simulink model "Model_TranslationEngine64"  (R2022b)
settings: Solver=FixedStepDiscrete  StartTime=0.0  StopTime=5  RelTol=1e-3  EnableMultiTasking=on
InitFcn:
  | % Initialize model
  | ModelSettings=BTConfig.GetModelSettings();
  | 
  | ModelSettings.Validate();
  | 
  | ModelInit;
  | 
  | 
  | % load library data
  | GainLibrary_data;
  | % Load saved values from partition process
  | CapturedConstMask.LoadMapFromFile(bdroot)
StartFcn:
  | % make sure all the simulated RTC requests are found
  | %RTC_SIM_OBJ.ValidateREQs();
undefined symbols (not defined in the file or in its folder): AA, BPLP, Column, NumHFRefBPF, NumHFRefLPF, NumMusicChannels, Row, VolumeMuteConfig
libraries: TuneVar x925, TOP x490, FeaturePath x111, CapturedConstLib x52
(part 16 of 34)

== system Model_TranslationEngine64/NEAR/Near1p1/VolumeMute/VolMuteCh2/Mute/MuteControl ==
  FeaturePath : FeaturePath/FeaturePath  FeatureName=Ann2Mute  IsGroup=off  GroupNumber=-1  IsModule=off  TriggerInit=[180 39 295 146]
      settings: SourceProductName=Bose Talaria
  TuneVarRampTime : Subsystem  Description=|  mask(Talaria Trivial Tune TOP){TriggerInit=[295 232 465 288], TopName=RampTime, TuneName=RampTime, DataTypeOut=single, MaskValue=Config.DefaultRampTimeMsec, TunabilityNumber=1, MinValue=1, MaxValue=100000, BankNumber=0, PreOverlay=false, PostOverlay=false, UseSameName=on}
      | Specifies the default value of ramp time for the Mute or Unmute operation.
      | Used only when the RTC message does not contain either ramp rate or ramp time.
      mask prompts: TriggerInit "Hidden: MoveFcn redraw"; TopName "Name:"; TuneName "Name of TuneVar:"; DataTypeOut "Data type:"; MaskValue "Default Value:"; TunabilityNumber "Tunability:"; MinValue "Min Value:"; MaxValue "Max Value:"; BankNumber "Target memory bank number:"; PreOverlay "Requires pre-overlay action:"; PostOverlay "Requires post-overlay action:"; UseSameName "Use same name for tune variable and TOP"
      mask help: The TuneTOP block encapsultes a Target Overlay Parameter, a Tune Variable, and a Trivial Translation between them.
      mask init:
      | [ok,activeTopPath,activeTunePath] = TuneTOP_Mask.Init(gcbh);
      settings: MoveFcn=TuneTOP_Mask.CB_TriggerInit(gcbh);
      mask Callback TriggerInit: TuneTOP_Mask.CB_TriggerInit(gcbh);
      mask TypeOptions TopName: TOP/TopName
      mask TypeOptions TuneName: Tune Variable/TuneName
      mask TypeOptions DataTypeOut: TOP/DataTypeOut
      mask TypeOptions MaskValue: Tune Variable/MaskValue
      mask TypeOptions TunabilityNumber: Tune Variable/TunabilityNumber
      mask Callback TunabilityNumber: TuneVarMask.CB_TunabilityNumber(gcbh);
      mask TypeOptions MinValue: Tune Variable/MinValue
      mask TypeOptions MaxValue: Tune Variable/MaxValue
      mask TypeOptions BankNumber: TOP/BankNumber
      mask TypeOptions PreOverlay: TOP/PreOverlay
      mask TypeOptions PostOverlay: TOP/PostOverlay
      mask Callback UseSameName: TuneTOP_Mask.CB_UseSameName(gcbh);
      mask DialogControl toolPanel Prompt: Tuning Tool Hints
      mask DialogControl DescriptionGroup Prompt: Description
      mask DialogControl EditDescription Prompt: Edit Description
      mask DialogControl EditDescription Callback: TuneTOP_Mask.CB_EditDescription(gcbh);
      mask DialogControl TunabilityText Prompt: Easy: Changes nearly every tuning.
      mask DialogControl AdvancedPanel Prompt: Advanced
      mask DialogControl ConvertToFullTranslation Prompt: Irreversible conversion to full translation
      mask DialogControl ConvertToFullTranslation Callback: TuneTOP_Mask.CB_ConvertToFullTranslation(gcbh);
      mask DialogControl ErrorContainer Prompt: Error Messages
      mask Display:
      | % retrieve icon definition
      | [path,w,h] = TuneTOP_Mask.Icon();
      | 
      | % retrieve the block's pixel size
      | pos = get(gcbh,'position');
      | bw = pos(3) - pos(1);
      | bh = pos(4) - pos(2);
      | 
      | % draw centered icon
      | xAdj = bw/2 - w/2 + 5;
      | yAdj = bh/2 - h/2 + 4;
      | for i=1:length(path)
      | 	patch(path(i).x+xAdj, path(i).y+yAdj, path(i).rgb);
      | end
      | 
      | % show the top name or an X
      | if (exist('ok','var') && ok)
      | 	text(bw*0.5, bh*0.2, activeTopPath, 'horizontalAlignment', 'center');
      | 	patch(0,0,[1 1 1]);
      | 	patch(bw,bh,[1 1 1]);
      | else
      | 	tx=bw*0.03;
      | 	ty=bh*0.03;
      | 	patch([0 tx bw bw-tx], [ty 0 bh-ty bh], [1 0 0]);
      | 	patch([0 bw-tx bw tx], [bh-ty 0 ty bh], [1 0 0]);
      | end

== system Model_TranslationEngine64/NEAR/Near1p1/VolumeMute/VolMuteCh2/Volume/TuneVarRampRate ==
  TOP : TOP/TOP  TriggerInit=[440 20 585 80]  TopName=RampRate  DataTypeOut=single  BankNumber=BankNumber  PreOverlay=PreOverlay  PostOverlay=PostOverlay  Role=Automatic
      settings: SourceProductName=Bose Talaria
  TrivialTranslation : TuneVar/TrivialTranslation  TriggerInit=[300 28 350 72]
      settings: SourceProductName=Bose Talaria
  Tune Variable : TuneVar/TuneVar  TuneName=RampRate  SpecifyMaxSize=off  VariableDim=1 (Row)  MaxSize=[1 1]  TunabilityNumber=2  MinValue=MinValue  MaxValue=MaxValue  TriggerInit=[20 25 190 75]  MaskValue=MaskValue
      settings: SourceProductName=Bose Talaria
  wires:
  Tune Variable/1 -> TrivialTranslation/1  "RampRate"
  TrivialTranslation/1 -> TOP/1

== system Model_TranslationEngine64/NEAR/Near1p1/VolumeMute/VolMuteCh2/Volume/TuneVarRampTime ==
  TOP : TOP/TOP  TriggerInit=[440 20 585 80]  TopName=RampTime  DataTypeOut=single  BankNumber=BankNumber  PreOverlay=PreOverlay  PostOverlay=PostOverlay  Role=Automatic
      settings: SourceProductName=Bose Talaria
  TrivialTranslation : TuneVar/TrivialTranslation  TriggerInit=[300 28 350 72]
      settings: SourceProductName=Bose Talaria
  Tune Variable : TuneVar/TuneVar  TuneName=RampTime  SpecifyMaxSize=off  VariableDim=1 (Row)  MaxSize=[1 1]  TunabilityNumber=1  MinValue=MinValue  MaxValue=MaxValue  TriggerInit=[20 25 190 75]  MaskValue=MaskValue
      settings: SourceProductName=Bose Talaria
  wires:
  Tune Variable/1 -> TrivialTranslation/1  "RampTime"
  TrivialTranslation/1 -> TOP/1

== system Model_TranslationEngine64/NEAR/Near1p1/VolumeMute/VolMuteCh3/Ann3NonEntGainCalc/TuneTOP ==
  TOP : TOP/TOP  TriggerInit=[440 20 585 80]  TopName=VncThresh  DataTypeOut=single  BankNumber=BankNumber  PreOverlay=PreOverlay  PostOverlay=PostOverlay  Role=Automatic
      settings: SourceProductName=Bose Talaria
  TrivialTranslation : TuneVar/TrivialTranslation  TriggerInit=[300 28 350 72]
      settings: SourceProductName=Bose Talaria
  Tune Variable : TuneVar/TuneVar  TuneName=VncThresh  SpecifyMaxSize=off  VariableDim=1 (Row)  MaxSize=[1 1]  TunabilityNumber=1  MinValue=MinValue  MaxValue=MaxValue  TriggerInit=[20 25 190 75]  MaskValue=MaskValue
      settings: SourceProductName=Bose Talaria
  wires:
  Tune Variable/1 -> TrivialTranslation/1  "VncThresh"
  TrivialTranslation/1 -> TOP/1

== system Model_TranslationEngine64/NEAR/Near1p1/VolumeMute/VolMuteCh3/Ann3NonEntGainCalc/TuneTOP1 ==
  TOP : TOP/TOP  TriggerInit=[440 20 585 80]  TopName=VncSlope  DataTypeOut=single  BankNumber=BankNumber  PreOverlay=PreOverlay  PostOverlay=PostOverlay  Role=Automatic
      settings: SourceProductName=Bose Talaria
  TrivialTranslation : TuneVar/TrivialTranslation  TriggerInit=[300 28 350 72]
      settings: SourceProductName=Bose Talaria
  Tune Variable : TuneVar/TuneVar  TuneName=VncSlope  SpecifyMaxSize=off  VariableDim=1 (Row)  MaxSize=[1 1]  TunabilityNumber=1  MinValue=MinValue  MaxValue=MaxValue  TriggerInit=[20 25 190 75]  MaskValue=MaskValue
      settings: SourceProductName=Bose Talaria
  wires:
  Tune Variable/1 -> TrivialTranslation/1  "VncSlope"
  TrivialTranslation/1 -> TOP/1

== system Model_TranslationEngine64/NEAR/Near1p1/VolumeMute/VolMuteCh3/Ann3NonEntGainCalc/TuneTOP2 ==
  TOP : TOP/TOP  TriggerInit=[440 20 585 80]  TopName=MaxBoost  DataTypeOut=single  BankNumber=BankNumber  PreOverlay=PreOverlay  PostOverlay=PostOverlay  Role=Automatic
      settings: SourceProductName=Bose Talaria
  TrivialTranslation : TuneVar/TrivialTranslation  TriggerInit=[300 28 350 72]
      settings: SourceProductName=Bose Talaria
  Tune Variable : TuneVar/TuneVar  TuneName=MaxBoost  SpecifyMaxSize=off  VariableDim=1 (Row)  MaxSize=[1 1]  TunabilityNumber=1  MinValue=MinValue  MaxValue=MaxValue  TriggerInit=[20 25 190 75]  MaskValue=MaskValue
      settings: SourceProductName=Bose Talaria
  wires:
  Tune Variable/1 -> TrivialTranslation/1  "MaxBoost"
  TrivialTranslation/1 -> TOP/1

== system Model_TranslationEngine64/NEAR/Near1p1/VolumeMute/VolMuteCh3/Ann3NonEntGainCalc/TuneTOP3 ==
  TOP : TOP/TOP  TriggerInit=[440 20 585 80]  TopName=NoiseOverRide  DataTypeOut=single  BankNumber=BankNumber  PreOverlay=PreOverlay  PostOverlay=PostOverlay  Role=Automatic
      settings: SourceProductName=Bose Talaria
  TrivialTranslation : TuneVar/TrivialTranslation  TriggerInit=[300 28 350 72]
      settings: SourceProductName=Bose Talaria
  Tune Variable : TuneVar/TuneVar  TuneName=NoiseOverRide  SpecifyMaxSize=off  VariableDim=1 (Row)  MaxSize=[1 1]  TunabilityNumber=1  MinValue=MinValue  MaxValue=MaxValue  TriggerInit=[20 25 190 75]  MaskValue=MaskValue
      settings: SourceProductName=Bose Talaria
  wires:
  Tune Variable/1 -> TrivialTranslation/1  "NoiseOverRide"
  TrivialTranslation/1 -> TOP/1

== system Model_TranslationEngine64/NEAR/Near1p1/VolumeMute/VolMuteCh3/Ann3NonEntGainCalc/TuneTOP4 ==
  TOP : TOP/TOP  TriggerInit=[440 20 585 80]  TopName=NoiseOverRideFlag  DataTypeOut=single  BankNumber=BankNumber  PreOverlay=PreOverlay  PostOverlay=PostOverlay  Role=Automatic
      settings: SourceProductName=Bose Talaria
  TrivialTranslation : TuneVar/TrivialTranslation  TriggerInit=[300 28 350 72]
      settings: SourceProductName=Bose Talaria
  Tune Variable : TuneVar/TuneVar  TuneName=NoiseOverRideFlag  SpecifyMaxSize=off  VariableDim=1 (Row)  MaxSize=[1 1]  TunabilityNumber=1  MinValue=MinValue  MaxValue=MaxValue  TriggerInit=[20 25 190 75]  MaskValue=MaskValue
      settings: SourceProductName=Bose Talaria
  wires:
  Tune Variable/1 -> TrivialTranslation/1  "NoiseOverRideFlag"
  TrivialTranslation/1 -> TOP/1

== system Model_TranslationEngine64/NEAR/Near1p1/VolumeMute/VolMuteCh3/Ann3NonEntGainCalc/TuneTOP5 ==
  TOP : TOP/TOP  TriggerInit=[440 20 585 80]  TopName=BoostOverRide  DataTypeOut=single  BankNumber=BankNumber  PreOverlay=PreOverlay  PostOverlay=PostOverlay  Role=Automatic
      settings: SourceProductName=Bose Talaria
  TrivialTranslation : TuneVar/TrivialTranslation  TriggerInit=[300 28 350 72]
      settings: SourceProductName=Bose Talaria
  Tune Variable : TuneVar/TuneVar  TuneName=BoostOverRide  SpecifyMaxSize=off  VariableDim=1 (Row)  MaxSize=[1 1]  TunabilityNumber=1  MinValue=MinValue  MaxValue=MaxValue  TriggerInit=[20 25 190 75]  MaskValue=MaskValue
      settings: SourceProductName=Bose Talaria
  wires:
  Tune Variable/1 -> TrivialTranslation/1  "BoostOverRide"
  TrivialTranslation/1 -> TOP/1

== system Model_TranslationEngine64/NEAR/Near1p1/VolumeMute/VolMuteCh3/Ann3NonEntGainCalc/TuneTOP6 ==
  TOP : TOP/TOP  TriggerInit=[440 20 585 80]  TopName=BoostOverRideFlag  DataTypeOut=single  BankNumber=BankNumber  PreOverlay=PreOverlay  PostOverlay=PostOverlay  Role=Automatic
      settings: SourceProductName=Bose Talaria
  TrivialTranslation : TuneVar/TrivialTranslation  TriggerInit=[300 28 350 72]
      settings: SourceProductName=Bose Talaria
  Tune Variable : TuneVar/TuneVar  TuneName=BoostOverRideFlag  SpecifyMaxSize=off  VariableDim=1 (Row)  MaxSize=[1 1]  TunabilityNumber=1  MinValue=MinValue  MaxValue=MaxValue  TriggerInit=[20 25 190 75]  MaskValue=MaskValue
      settings: SourceProductName=Bose Talaria
  wires:
  Tune Variable/1 -> TrivialTranslation/1  "BoostOverRideFlag"
  TrivialTranslation/1 -> TOP/1

== system Model_TranslationEngine64/NEAR/Near1p1/VolumeMute/VolMuteCh3/Ann3NonEntGainCalc/TuneTOP7 ==
  TOP : TOP/TOP  TriggerInit=[440 20 585 80]  TopName=VncEnableTuneVar  DataTypeOut=single  BankNumber=BankNumber  PreOverlay=PreOverlay  PostOverlay=PostOverlay  Role=Automatic
      settings: SourceProductName=Bose Talaria
  TrivialTranslation : TuneVar/TrivialTranslation  TriggerInit=[300 28 350 72]
      settings: SourceProductName=Bose Talaria
  Tune Variable : TuneVar/TuneVar  TuneName=VncEnableTuneVar  SpecifyMaxSize=off  VariableDim=1 (Row)  MaxSize=[1 1]  TunabilityNumber=1  MinValue=MinValue  MaxValue=MaxValue  TriggerInit=[20 25 190 75]  MaskValue=MaskValue
      settings: SourceProductName=Bose Talaria
  wires:
  Tune Variable/1 -> TrivialTranslation/1  "VncEnableTuneVar"
  TrivialTranslation/1 -> TOP/1

== system Model_TranslationEngine64/NEAR/Near1p1/VolumeMute/VolMuteCh3/Ann3NonEntGainCalc/TuneTOP8 ==
  TranslateTrigger : TuneVar/TranslateTrigger  TriggerInit=[306 -100 344 -45]
      settings: SourceProductName=Bose Talaria
  den : TOP/TOP  TriggerInit=[450 90 595 150]  TopName=Den  DataTypeOut=single  BankNumber=0  PreOverlay=false  PostOverlay=false  Role=Automatic
      settings: SourceProductName=Bose Talaria
  num : TOP/TOP  TriggerInit=[450 -45 595 15]  TopName=Num  DataTypeOut=single  BankNumber=0  PreOverlay=false  PostOverlay=false  Role=Automatic
      settings: SourceProductName=Bose Talaria
  translation : MATLAB Function  TreatAsAtomicUnit=on  mask{L=Config.FrameSize, Fd=Config.Fd}
  tuneVARTau : TuneVar/TuneVar  TuneName=Tau  SpecifyMaxSize=off  VariableDim=1 (Row)  MaxSize=[1 1]  TunabilityNumber=1  MinValue=[]  MaxValue=[]  TriggerInit=[-70 25 100 75]  MaskValue=Config.DefaultTau
      settings: SourceProductName=Bose Talaria
  wires:
  tuneVARTau/1 -> translation/1(tau)  "Tau"
  TranslateTrigger/1 -> translation/Trigger
  translation/2(Den) -> den/1
  translation/1(Num) -> num/1

== system Model_TranslationEngine64/NEAR/Near1p1/VolumeMute/VolMuteCh3/Ann3NonEntGainCalc/vncSignal ==
  TuneTOP : Subsystem  mask(Talaria Trivial Tune TOP){TriggerInit=[50 -8 220 48], TopName=MinVncSignal, TuneName=MinVncSignal, DataTypeOut=single, MaskValue=Config.DefaultMinVncSignal, TunabilityNumber=1, MinValue=[], MaxValue=[], BankNumber=0, PreOverlay=false, PostOverlay=false, UseSameName=on}
      mask prompts: TriggerInit "Hidden: MoveFcn redraw"; TopName "Name:"; TuneName "Name of TuneVar:"; DataTypeOut "Data type:"; MaskValue "Default Value:"; TunabilityNumber "Tunability:"; MinValue "Min Value:"; MaxValue "Max Value:"; BankNumber "Target memory bank number:"; PreOverlay "Requires pre-overlay action:"; PostOverlay "Requires post-overlay action:"; UseSameName "Use same name for tune variable and TOP"
      mask help: The TuneTOP block encapsultes a Target Overlay Parameter, a Tune Variable, and a Trivial Translation between them.
      mask init:
      | [ok,activeTopPath,activeTunePath] = TuneTOP_Mask.Init(gcbh);
      settings: MoveFcn=TuneTOP_Mask.CB_TriggerInit(gcbh);
      mask Callback TriggerInit: TuneTOP_Mask.CB_TriggerInit(gcbh);
      mask TypeOptions TopName: TOP/TopName
      mask TypeOptions TuneName: Tune Variable/TuneName
      mask TypeOptions DataTypeOut: TOP/DataTypeOut
      mask TypeOptions MaskValue: Tune Variable/MaskValue
      mask TypeOptions TunabilityNumber: Tune Variable/TunabilityNumber
      mask Callback TunabilityNumber: TuneVarMask.CB_TunabilityNumber(gcbh);
      mask TypeOptions MinValue: Tune Variable/MinValue
      mask TypeOptions MaxValue: Tune Variable/MaxValue
      mask TypeOptions BankNumber: TOP/BankNumber
      mask TypeOptions PreOverlay: TOP/PreOverlay
      mask TypeOptions PostOverlay: TOP/PostOverlay
      mask Callback UseSameName: TuneTOP_Mask.CB_UseSameName(gcbh);
      mask DialogControl toolPanel Prompt: Tuning Tool Hints
      mask DialogControl DescriptionGroup Prompt: Description
      mask DialogControl EditDescription Prompt: Edit Description
      mask DialogControl EditDescription Callback: TuneTOP_Mask.CB_EditDescription(gcbh);
      mask DialogControl TunabilityText Prompt: Easy: Changes nearly every tuning.
      mask DialogControl AdvancedPanel Prompt: Advanced
      mask DialogControl ConvertToFullTranslation Prompt: Irreversible conversion to full translation
      mask DialogControl ConvertToFullTranslation Callback: TuneTOP_Mask.CB_ConvertToFullTranslation(gcbh);
      mask DialogControl ErrorContainer Prompt: Error Messages
      mask Display:
      | % retrieve icon definition
      | [path,w,h] = TuneTOP_Mask.Icon();
      | 
      | % retrieve the block's pixel size
      | pos = get(gcbh,'position');
      | bw = pos(3) - pos(1);
      | bh = pos(4) - pos(2);
      | 
      | % draw centered icon
      | xAdj = bw/2 - w/2 + 5;
      | yAdj = bh/2 - h/2 + 4;
      | for i=1:length(path)
      | 	patch(path(i).x+xAdj, path(i).y+yAdj, path(i).rgb);
      | end
      | 
      | % show the top name or an X
      | if (exist('ok','var') && ok)
      | 	text(bw*0.5, bh*0.2, activeTopPath, 'horizontalAlignment', 'center');
      | 	patch(0,0,[1 1 1]);
      | 	patch(bw,bh,[1 1 1]);
      | else
      | 	tx=bw*0.03;
      | 	ty=bh*0.03;
      | 	patch([0 tx bw bw-tx], [ty 0 bh-ty bh], [1 0 0]);
      | 	patch([0 bw-tx bw tx], [bh-ty 0 ty bh], [1 0 0]);
      | end
  TuneTOP1 : Subsystem  mask(Talaria Trivial Tune TOP){TriggerInit=[40 142 210 198], TopName=MaxSpl, TuneName=MaxSpl, DataTypeOut=single, MaskValue=Config.DefaultMaxSpl, TunabilityNumber=1, MinValue=[], MaxValue=[], BankNumber=0, PreOverlay=false, PostOverlay=false, UseSameName=on}
      mask prompts: TriggerInit "Hidden: MoveFcn redraw"; TopName "Name:"; TuneName "Name of TuneVar:"; DataTypeOut "Data type:"; MaskValue "Default Value:"; TunabilityNumber "Tunability:"; MinValue "Min Value:"; MaxValue "Max Value:"; BankNumber "Target memory bank number:"; PreOverlay "Requires pre-overlay action:"; PostOverlay "Requires post-overlay action:"; UseSameName "Use same name for tune variable and TOP"
      mask help: The TuneTOP block encapsultes a Target Overlay Parameter, a Tune Variable, and a Trivial Translation between them.
      mask init:
      | [ok,activeTopPath,activeTunePath] = TuneTOP_Mask.Init(gcbh);
      settings: MoveFcn=TuneTOP_Mask.CB_TriggerInit(gcbh);
      mask Callback TriggerInit: TuneTOP_Mask.CB_TriggerInit(gcbh);
      mask TypeOptions TopName: TOP/TopName
      mask TypeOptions TuneName: Tune Variable/TuneName
      mask TypeOptions DataTypeOut: TOP/DataTypeOut
      mask TypeOptions MaskValue: Tune Variable/MaskValue
      mask TypeOptions TunabilityNumber: Tune Variable/TunabilityNumber
      mask Callback TunabilityNumber: TuneVarMask.CB_TunabilityNumber(gcbh);
      mask TypeOptions MinValue: Tune Variable/MinValue
      mask TypeOptions MaxValue: Tune Variable/MaxValue
      mask TypeOptions BankNumber: TOP/BankNumber
      mask TypeOptions PreOverlay: TOP/PreOverlay
      mask TypeOptions PostOverlay: TOP/PostOverlay
      mask Callback UseSameName: TuneTOP_Mask.CB_UseSameName(gcbh);
      mask DialogControl toolPanel Prompt: Tuning Tool Hints
      mask DialogControl DescriptionGroup Prompt: Description
      mask DialogControl EditDescription Prompt: Edit Description
      mask DialogControl EditDescription Callback: TuneTOP_Mask.CB_EditDescription(gcbh);
      mask DialogControl TunabilityText Prompt: Easy: Changes nearly every tuning.
      mask DialogControl AdvancedPanel Prompt: Advanced
      mask DialogControl ConvertToFullTranslation Prompt: Irreversible conversion to full translation
      mask DialogControl ConvertToFullTranslation Callback: TuneTOP_Mask.CB_ConvertToFullTranslation(gcbh);
      mask DialogControl ErrorContainer Prompt: Error Messages
      mask Display:
      | % retrieve icon definition
      | [path,w,h] = TuneTOP_Mask.Icon();
      | 
      | % retrieve the block's pixel size
      | pos = get(gcbh,'position');
      | bw = pos(3) - pos(1);
      | bh = pos(4) - pos(2);
      | 
      | % draw centered icon
      | xAdj = bw/2 - w/2 + 5;
      | yAdj = bh/2 - h/2 + 4;
      | for i=1:length(path)
      | 	patch(path(i).x+xAdj, path(i).y+yAdj, path(i).rgb);
      | end
      | 
      | % show the top name or an X
      | if (exist('ok','var') && ok)
      | 	text(bw*0.5, bh*0.2, activeTopPath, 'horizontalAlignment', 'center');
      | 	patch(0,0,[1 1 1]);
      | 	patch(bw,bh,[1 1 1]);
      | else
      | 	tx=bw*0.03;
      | 	ty=bh*0.03;
      | 	patch([0 tx bw bw-tx], [ty 0 bh-ty bh], [1 0 0]);
      | 	patch([0 bw-tx bw tx], [bh-ty 0 ty bh], [1 0 0]);
      | end

== system Model_TranslationEngine64/NEAR/Near1p1/VolumeMute/VolMuteCh3/Ann3NonEntVncApplied/nonentVNCApplied_subsystem ==
  TuneTOP : Subsystem

== system Model_TranslationEngine64/NEAR/Near1p1/VolumeMute/VolMuteCh3/Mute/MuteControl ==
  FeaturePath : FeaturePath/FeaturePath  FeatureName=Ann3Mute  IsGroup=off  GroupNumber=-1  IsModule=off  TriggerInit=[180 39 295 146]
      settings: SourceProductName=Bose Talaria
  TuneVarRampTime : Subsystem  Description=|  mask(Talaria Trivial Tune TOP){TriggerInit=[295 232 465 288], TopName=RampTime, TuneName=RampTime, DataTypeOut=single, MaskValue=Config.DefaultRampTimeMsec, TunabilityNumber=1, MinValue=1, MaxValue=100000, BankNumber=0, PreOverlay=false, PostOverlay=false, UseSameName=on}
      | Specifies the default value of ramp time for the Mute or Unmute operation.
      | Used only when the RTC message does not contain either ramp rate or ramp time.
      mask prompts: TriggerInit "Hidden: MoveFcn redraw"; TopName "Name:"; TuneName "Name of TuneVar:"; DataTypeOut "Data type:"; MaskValue "Default Value:"; TunabilityNumber "Tunability:"; MinValue "Min Value:"; MaxValue "Max Value:"; BankNumber "Target memory bank number:"; PreOverlay "Requires pre-overlay action:"; PostOverlay "Requires post-overlay action:"; UseSameName "Use same name for tune variable and TOP"
      mask help: The TuneTOP block encapsultes a Target Overlay Parameter, a Tune Variable, and a Trivial Translation between them.
      mask init:
      | [ok,activeTopPath,activeTunePath] = TuneTOP_Mask.Init(gcbh);
      settings: MoveFcn=TuneTOP_Mask.CB_TriggerInit(gcbh);
      mask Callback TriggerInit: TuneTOP_Mask.CB_TriggerInit(gcbh);
      mask TypeOptions TopName: TOP/TopName
      mask TypeOptions TuneName: Tune Variable/TuneName
      mask TypeOptions DataTypeOut: TOP/DataTypeOut
      mask TypeOptions MaskValue: Tune Variable/MaskValue
      mask TypeOptions TunabilityNumber: Tune Variable/TunabilityNumber
      mask Callback TunabilityNumber: TuneVarMask.CB_TunabilityNumber(gcbh);
      mask TypeOptions MinValue: Tune Variable/MinValue
      mask TypeOptions MaxValue: Tune Variable/MaxValue
      mask TypeOptions BankNumber: TOP/BankNumber
      mask TypeOptions PreOverlay: TOP/PreOverlay
      mask TypeOptions PostOverlay: TOP/PostOverlay
      mask Callback UseSameName: TuneTOP_Mask.CB_UseSameName(gcbh);
      mask DialogControl toolPanel Prompt: Tuning Tool Hints
      mask DialogControl DescriptionGroup Prompt: Description
      mask DialogControl EditDescription Prompt: Edit Description
      mask DialogControl EditDescription Callback: TuneTOP_Mask.CB_EditDescription(gcbh);
      mask DialogControl TunabilityText Prompt: Easy: Changes nearly every tuning.
      mask DialogControl AdvancedPanel Prompt: Advanced
      mask DialogControl ConvertToFullTranslation Prompt: Irreversible conversion to full translation
      mask DialogControl ConvertToFullTranslation Callback: TuneTOP_Mask.CB_ConvertToFullTranslation(gcbh);
      mask DialogControl ErrorContainer Prompt: Error Messages
      mask Display:
      | % retrieve icon definition
      | [path,w,h] = TuneTOP_Mask.Icon();
      | 
      | % retrieve the block's pixel size
      | pos = get(gcbh,'position');
      | bw = pos(3) - pos(1);
      | bh = pos(4) - pos(2);
      | 
      | % draw centered icon
      | xAdj = bw/2 - w/2 + 5;
      | yAdj = bh/2 - h/2 + 4;
      | for i=1:length(path)
      | 	patch(path(i).x+xAdj, path(i).y+yAdj, path(i).rgb);
      | end
      | 
      | % show the top name or an X
      | if (exist('ok','var') && ok)
      | 	text(bw*0.5, bh*0.2, activeTopPath, 'horizontalAlignment', 'center');
      | 	patch(0,0,[1 1 1]);
      | 	patch(bw,bh,[1 1 1]);
      | else
      | 	tx=bw*0.03;
      | 	ty=bh*0.03;
      | 	patch([0 tx bw bw-tx], [ty 0 bh-ty bh], [1 0 0]);
      | 	patch([0 bw-tx bw tx], [bh-ty 0 ty bh], [1 0 0]);
      | end

== system Model_TranslationEngine64/NEAR/Near1p1/VolumeMute/VolMuteCh3/Volume/TuneVarRampRate ==
  TOP : TOP/TOP  TriggerInit=[440 20 585 80]  TopName=RampRate  DataTypeOut=single  BankNumber=BankNumber  PreOverlay=PreOverlay  PostOverlay=PostOverlay  Role=Automatic
      settings: SourceProductName=Bose Talaria
  TrivialTranslation : TuneVar/TrivialTranslation  TriggerInit=[300 28 350 72]
      settings: SourceProductName=Bose Talaria
  Tune Variable : TuneVar/TuneVar  TuneName=RampRate  SpecifyMaxSize=off  VariableDim=1 (Row)  MaxSize=[1 1]  TunabilityNumber=2  MinValue=MinValue  MaxValue=MaxValue  TriggerInit=[20 25 190 75]  MaskValue=MaskValue
      settings: SourceProductName=Bose Talaria
  wires:
  Tune Variable/1 -> TrivialTranslation/1  "RampRate"
  TrivialTranslation/1 -> TOP/1

== system Model_TranslationEngine64/NEAR/Near1p1/VolumeMute/VolMuteCh3/Volume/TuneVarRampTime ==
  TOP : TOP/TOP  TriggerInit=[440 20 585 80]  TopName=RampTime  DataTypeOut=single  BankNumber=BankNumber  PreOverlay=PreOverlay  PostOverlay=PostOverlay  Role=Automatic
      settings: SourceProductName=Bose Talaria
  TrivialTranslation : TuneVar/TrivialTranslation  TriggerInit=[300 28 350 72]
      settings: SourceProductName=Bose Talaria
  Tune Variable : TuneVar/TuneVar  TuneName=RampTime  SpecifyMaxSize=off  VariableDim=1 (Row)  MaxSize=[1 1]  TunabilityNumber=1  MinValue=MinValue  MaxValue=MaxValue  TriggerInit=[20 25 190 75]  MaskValue=MaskValue
      settings: SourceProductName=Bose Talaria
  wires:
  Tune Variable/1 -> TrivialTranslation/1  "RampTime"
  TrivialTranslation/1 -> TOP/1

== system Model_TranslationEngine64/NEAR/Near1p1/VolumeMute/VolMuteCh4/Ann4NonEntGainCalc/TuneTOP ==
  TOP : TOP/TOP  TriggerInit=[440 20 585 80]  TopName=VncThresh  DataTypeOut=single  BankNumber=BankNumber  PreOverlay=PreOverlay  PostOverlay=PostOverlay  Role=Automatic
      settings: SourceProductName=Bose Talaria
  TrivialTranslation : TuneVar/TrivialTranslation  TriggerInit=[300 28 350 72]
      settings: SourceProductName=Bose Talaria
  Tune Variable : TuneVar/TuneVar  TuneName=VncThresh  SpecifyMaxSize=off  VariableDim=1 (Row)  MaxSize=[1 1]  TunabilityNumber=1  MinValue=MinValue  MaxValue=MaxValue  TriggerInit=[20 25 190 75]  MaskValue=MaskValue
      settings: SourceProductName=Bose Talaria
  wires:
  Tune Variable/1 -> TrivialTranslation/1  "VncThresh"
  TrivialTranslation/1 -> TOP/1

== system Model_TranslationEngine64/NEAR/Near1p1/VolumeMute/VolMuteCh4/Ann4NonEntGainCalc/TuneTOP1 ==
  TOP : TOP/TOP  TriggerInit=[440 20 585 80]  TopName=VncSlope  DataTypeOut=single  BankNumber=BankNumber  PreOverlay=PreOverlay  PostOverlay=PostOverlay  Role=Automatic
      settings: SourceProductName=Bose Talaria
  TrivialTranslation : TuneVar/TrivialTranslation  TriggerInit=[300 28 350 72]
      settings: SourceProductName=Bose Talaria
  Tune Variable : TuneVar/TuneVar  TuneName=VncSlope  SpecifyMaxSize=off  VariableDim=1 (Row)  MaxSize=[1 1]  TunabilityNumber=1  MinValue=MinValue  MaxValue=MaxValue  TriggerInit=[20 25 190 75]  MaskValue=MaskValue
      settings: SourceProductName=Bose Talaria
  wires:
  Tune Variable/1 -> TrivialTranslation/1  "VncSlope"
  TrivialTranslation/1 -> TOP/1

== system Model_TranslationEngine64/NEAR/Near1p1/VolumeMute/VolMuteCh4/Ann4NonEntGainCalc/TuneTOP2 ==
  TOP : TOP/TOP  TriggerInit=[440 20 585 80]  TopName=MaxBoost  DataTypeOut=single  BankNumber=BankNumber  PreOverlay=PreOverlay  PostOverlay=PostOverlay  Role=Automatic
      settings: SourceProductName=Bose Talaria
  TrivialTranslation : TuneVar/TrivialTranslation  TriggerInit=[300 28 350 72]
      settings: SourceProductName=Bose Talaria
  Tune Variable : TuneVar/TuneVar  TuneName=MaxBoost  SpecifyMaxSize=off  VariableDim=1 (Row)  MaxSize=[1 1]  TunabilityNumber=1  MinValue=MinValue  MaxValue=MaxValue  TriggerInit=[20 25 190 75]  MaskValue=MaskValue
      settings: SourceProductName=Bose Talaria
  wires:
  Tune Variable/1 -> TrivialTranslation/1  "MaxBoost"
  TrivialTranslation/1 -> TOP/1

== system Model_TranslationEngine64/NEAR/Near1p1/VolumeMute/VolMuteCh4/Ann4NonEntGainCalc/TuneTOP3 ==
  TOP : TOP/TOP  TriggerInit=[440 20 585 80]  TopName=NoiseOverRide  DataTypeOut=single  BankNumber=BankNumber  PreOverlay=PreOverlay  PostOverlay=PostOverlay  Role=Automatic
      settings: SourceProductName=Bose Talaria
  TrivialTranslation : TuneVar/TrivialTranslation  TriggerInit=[300 28 350 72]
      settings: SourceProductName=Bose Talaria
  Tune Variable : TuneVar/TuneVar  TuneName=NoiseOverRide  SpecifyMaxSize=off  VariableDim=1 (Row)  MaxSize=[1 1]  TunabilityNumber=1  MinValue=MinValue  MaxValue=MaxValue  TriggerInit=[20 25 190 75]  MaskValue=MaskValue
      settings: SourceProductName=Bose Talaria
  wires:
  Tune Variable/1 -> TrivialTranslation/1  "NoiseOverRide"
  TrivialTranslation/1 -> TOP/1

== system Model_TranslationEngine64/NEAR/Near1p1/VolumeMute/VolMuteCh4/Ann4NonEntGainCalc/TuneTOP4 ==
  TOP : TOP/TOP  TriggerInit=[440 20 585 80]  TopName=NoiseOverRideFlag  DataTypeOut=single  BankNumber=BankNumber  PreOverlay=PreOverlay  PostOverlay=PostOverlay  Role=Automatic
      settings: SourceProductName=Bose Talaria
  TrivialTranslation : TuneVar/TrivialTranslation  TriggerInit=[300 28 350 72]
      settings: SourceProductName=Bose Talaria
  Tune Variable : TuneVar/TuneVar  TuneName=NoiseOverRideFlag  SpecifyMaxSize=off  VariableDim=1 (Row)  MaxSize=[1 1]  TunabilityNumber=1  MinValue=MinValue  MaxValue=MaxValue  TriggerInit=[20 25 190 75]  MaskValue=MaskValue
      settings: SourceProductName=Bose Talaria
  wires:
  Tune Variable/1 -> TrivialTranslation/1  "NoiseOverRideFlag"
  TrivialTranslation/1 -> TOP/1

== system Model_TranslationEngine64/NEAR/Near1p1/VolumeMute/VolMuteCh4/Ann4NonEntGainCalc/TuneTOP5 ==
  TOP : TOP/TOP  TriggerInit=[440 20 585 80]  TopName=BoostOverRide  DataTypeOut=single  BankNumber=BankNumber  PreOverlay=PreOverlay  PostOverlay=PostOverlay  Role=Automatic
      settings: SourceProductName=Bose Talaria
  TrivialTranslation : TuneVar/TrivialTranslation  TriggerInit=[300 28 350 72]
      settings: SourceProductName=Bose Talaria
  Tune Variable : TuneVar/TuneVar  TuneName=BoostOverRide  SpecifyMaxSize=off  VariableDim=1 (Row)  MaxSize=[1 1]  TunabilityNumber=1  MinValue=MinValue  MaxValue=MaxValue  TriggerInit=[20 25 190 75]  MaskValue=MaskValue
      settings: SourceProductName=Bose Talaria
  wires:
  Tune Variable/1 -> TrivialTranslation/1  "BoostOverRide"
  TrivialTranslation/1 -> TOP/1

== system Model_TranslationEngine64/NEAR/Near1p1/VolumeMute/VolMuteCh4/Ann4NonEntGainCalc/TuneTOP6 ==
  TOP : TOP/TOP  TriggerInit=[440 20 585 80]  TopName=BoostOverRideFlag  DataTypeOut=single  BankNumber=BankNumber  PreOverlay=PreOverlay  PostOverlay=PostOverlay  Role=Automatic
      settings: SourceProductName=Bose Talaria
  TrivialTranslation : TuneVar/TrivialTranslation  TriggerInit=[300 28 350 72]
      settings: SourceProductName=Bose Talaria
  Tune Variable : TuneVar/TuneVar  TuneName=BoostOverRideFlag  SpecifyMaxSize=off  VariableDim=1 (Row)  MaxSize=[1 1]  TunabilityNumber=1  MinValue=MinValue  MaxValue=MaxValue  TriggerInit=[20 25 190 75]  MaskValue=MaskValue
      settings: SourceProductName=Bose Talaria
  wires:
  Tune Variable/1 -> TrivialTranslation/1  "BoostOverRideFlag"
  TrivialTranslation/1 -> TOP/1

== system Model_TranslationEngine64/NEAR/Near1p1/VolumeMute/VolMuteCh4/Ann4NonEntGainCalc/TuneTOP7 ==
  TOP : TOP/TOP  TriggerInit=[440 20 585 80]  TopName=VncEnableTuneVar  DataTypeOut=single  BankNumber=BankNumber  PreOverlay=PreOverlay  PostOverlay=PostOverlay  Role=Automatic
      settings: SourceProductName=Bose Talaria
  TrivialTranslation : TuneVar/TrivialTranslation  TriggerInit=[300 28 350 72]
      settings: SourceProductName=Bose Talaria
  Tune Variable : TuneVar/TuneVar  TuneName=VncEnableTuneVar  SpecifyMaxSize=off  VariableDim=1 (Row)  MaxSize=[1 1]  TunabilityNumber=1  MinValue=MinValue  MaxValue=MaxValue  TriggerInit=[20 25 190 75]  MaskValue=MaskValue
      settings: SourceProductName=Bose Talaria
  wires:
  Tune Variable/1 -> TrivialTranslation/1  "VncEnableTuneVar"
  TrivialTranslation/1 -> TOP/1

== system Model_TranslationEngine64/NEAR/Near1p1/VolumeMute/VolMuteCh4/Ann4NonEntGainCalc/TuneTOP8 ==
  TranslateTrigger : TuneVar/TranslateTrigger  TriggerInit=[306 -100 344 -45]
      settings: SourceProductName=Bose Talaria
  den : TOP/TOP  TriggerInit=[450 90 595 150]  TopName=Den  DataTypeOut=single  BankNumber=0  PreOverlay=false  PostOverlay=false  Role=Automatic
      settings: SourceProductName=Bose Talaria
  num : TOP/TOP  TriggerInit=[450 -45 595 15]  TopName=Num  DataTypeOut=single  BankNumber=0  PreOverlay=false  PostOverlay=false  Role=Automatic
      settings: SourceProductName=Bose Talaria
  translation : MATLAB Function  TreatAsAtomicUnit=on  mask{L=Config.FrameSize, Fd=Config.Fd}
  tuneVARTau : TuneVar/TuneVar  TuneName=Tau  SpecifyMaxSize=off  VariableDim=1 (Row)  MaxSize=[1 1]  TunabilityNumber=1  MinValue=[]  MaxValue=[]  TriggerInit=[-70 25 100 75]  MaskValue=Config.DefaultTau
      settings: SourceProductName=Bose Talaria
  wires:
  tuneVARTau/1 -> translation/1(tau)  "Tau"
  TranslateTrigger/1 -> translation/Trigger
  translation/2(Den) -> den/1
  translation/1(Num) -> num/1

== system Model_TranslationEngine64/NEAR/Near1p1/VolumeMute/VolMuteCh4/Ann4NonEntGainCalc/vncSignal ==
  TuneTOP : Subsystem  mask(Talaria Trivial Tune TOP){TriggerInit=[50 -8 220 48], TopName=MinVncSignal, TuneName=MinVncSignal, DataTypeOut=single, MaskValue=Config.DefaultMinVncSignal, TunabilityNumber=1, MinValue=[], MaxValue=[], BankNumber=0, PreOverlay=false, PostOverlay=false, UseSameName=on}
      mask prompts: TriggerInit "Hidden: MoveFcn redraw"; TopName "Name:"; TuneName "Name of TuneVar:"; DataTypeOut "Data type:"; MaskValue "Default Value:"; TunabilityNumber "Tunability:"; MinValue "Min Value:"; MaxValue "Max Value:"; BankNumber "Target memory bank number:"; PreOverlay "Requires pre-overlay action:"; PostOverlay "Requires post-overlay action:"; UseSameName "Use same name for tune variable and TOP"
      mask help: The TuneTOP block encapsultes a Target Overlay Parameter, a Tune Variable, and a Trivial Translation between them.
      mask init:
      | [ok,activeTopPath,activeTunePath] = TuneTOP_Mask.Init(gcbh);
      settings: MoveFcn=TuneTOP_Mask.CB_TriggerInit(gcbh);
      mask Callback TriggerInit: TuneTOP_Mask.CB_TriggerInit(gcbh);
      mask TypeOptions TopName: TOP/TopName
      mask TypeOptions TuneName: Tune Variable/TuneName
      mask TypeOptions DataTypeOut: TOP/DataTypeOut
      mask TypeOptions MaskValue: Tune Variable/MaskValue
      mask TypeOptions TunabilityNumber: Tune Variable/TunabilityNumber
      mask Callback TunabilityNumber: TuneVarMask.CB_TunabilityNumber(gcbh);
      mask TypeOptions MinValue: Tune Variable/MinValue
      mask TypeOptions MaxValue: Tune Variable/MaxValue
      mask TypeOptions BankNumber: TOP/BankNumber
      mask TypeOptions PreOverlay: TOP/PreOverlay
      mask TypeOptions PostOverlay: TOP/PostOverlay
      mask Callback UseSameName: TuneTOP_Mask.CB_UseSameName(gcbh);
      mask DialogControl toolPanel Prompt: Tuning Tool Hints
      mask DialogControl DescriptionGroup Prompt: Description
      mask DialogControl EditDescription Prompt: Edit Description
      mask DialogControl EditDescription Callback: TuneTOP_Mask.CB_EditDescription(gcbh);
      mask DialogControl TunabilityText Prompt: Easy: Changes nearly every tuning.
      mask DialogControl AdvancedPanel Prompt: Advanced
      mask DialogControl ConvertToFullTranslation Prompt: Irreversible conversion to full translation
      mask DialogControl ConvertToFullTranslation Callback: TuneTOP_Mask.CB_ConvertToFullTranslation(gcbh);
      mask DialogControl ErrorContainer Prompt: Error Messages
      mask Display:
      | % retrieve icon definition
      | [path,w,h] = TuneTOP_Mask.Icon();
      | 
      | % retrieve the block's pixel size
      | pos = get(gcbh,'position');
      | bw = pos(3) - pos(1);
      | bh = pos(4) - pos(2);
      | 
      | % draw centered icon
      | xAdj = bw/2 - w/2 + 5;
      | yAdj = bh/2 - h/2 + 4;
      | for i=1:length(path)
      | 	patch(path(i).x+xAdj, path(i).y+yAdj, path(i).rgb);
      | end
      | 
      | % show the top name or an X
      | if (exist('ok','var') && ok)
      | 	text(bw*0.5, bh*0.2, activeTopPath, 'horizontalAlignment', 'center');
      | 	patch(0,0,[1 1 1]);
      | 	patch(bw,bh,[1 1 1]);
      | else
      | 	tx=bw*0.03;
      | 	ty=bh*0.03;
      | 	patch([0 tx bw bw-tx], [ty 0 bh-ty bh], [1 0 0]);
      | 	patch([0 bw-tx bw tx], [bh-ty 0 ty bh], [1 0 0]);
      | end
  TuneTOP1 : Subsystem  mask(Talaria Trivial Tune TOP){TriggerInit=[40 142 210 198], TopName=MaxSpl, TuneName=MaxSpl, DataTypeOut=single, MaskValue=Config.DefaultMaxSpl, TunabilityNumber=1, MinValue=[], MaxValue=[], BankNumber=0, PreOverlay=false, PostOverlay=false, UseSameName=on}
      mask prompts: TriggerInit "Hidden: MoveFcn redraw"; TopName "Name:"; TuneName "Name of TuneVar:"; DataTypeOut "Data type:"; MaskValue "Default Value:"; TunabilityNumber "Tunability:"; MinValue "Min Value:"; MaxValue "Max Value:"; BankNumber "Target memory bank number:"; PreOverlay "Requires pre-overlay action:"; PostOverlay "Requires post-overlay action:"; UseSameName "Use same name for tune variable and TOP"
      mask help: The TuneTOP block encapsultes a Target Overlay Parameter, a Tune Variable, and a Trivial Translation between them.
      mask init:
      | [ok,activeTopPath,activeTunePath] = TuneTOP_Mask.Init(gcbh);
      settings: MoveFcn=TuneTOP_Mask.CB_TriggerInit(gcbh);
      mask Callback TriggerInit: TuneTOP_Mask.CB_TriggerInit(gcbh);
      mask TypeOptions TopName: TOP/TopName
      mask TypeOptions TuneName: Tune Variable/TuneName
      mask TypeOptions DataTypeOut: TOP/DataTypeOut
      mask TypeOptions MaskValue: Tune Variable/MaskValue
      mask TypeOptions TunabilityNumber: Tune Variable/TunabilityNumber
      mask Callback TunabilityNumber: TuneVarMask.CB_TunabilityNumber(gcbh);
      mask TypeOptions MinValue: Tune Variable/MinValue
      mask TypeOptions MaxValue: Tune Variable/MaxValue
      mask TypeOptions BankNumber: TOP/BankNumber
      mask TypeOptions PreOverlay: TOP/PreOverlay
      mask TypeOptions PostOverlay: TOP/PostOverlay
      mask Callback UseSameName: TuneTOP_Mask.CB_UseSameName(gcbh);
      mask DialogControl toolPanel Prompt: Tuning Tool Hints
      mask DialogControl DescriptionGroup Prompt: Description
      mask DialogControl EditDescription Prompt: Edit Description
      mask DialogControl EditDescription Callback: TuneTOP_Mask.CB_EditDescription(gcbh);
      mask DialogControl TunabilityText Prompt: Easy: Changes nearly every tuning.
      mask DialogControl AdvancedPanel Prompt: Advanced
      mask DialogControl ConvertToFullTranslation Prompt: Irreversible conversion to full translation
      mask DialogControl ConvertToFullTranslation Callback: TuneTOP_Mask.CB_ConvertToFullTranslation(gcbh);
      mask DialogControl ErrorContainer Prompt: Error Messages
      mask Display:
      | % retrieve icon definition
      | [path,w,h] = TuneTOP_Mask.Icon();
      | 
      | % retrieve the block's pixel size
      | pos = get(gcbh,'position');
      | bw = pos(3) - pos(1);
      | bh = pos(4) - pos(2);
      | 
      | % draw centered icon
      | xAdj = bw/2 - w/2 + 5;
      | yAdj = bh/2 - h/2 + 4;
      | for i=1:length(path)
      | 	patch(path(i).x+xAdj, path(i).y+yAdj, path(i).rgb);
      | end
      | 
      | % show the top name or an X
      | if (exist('ok','var') && ok)
      | 	text(bw*0.5, bh*0.2, activeTopPath, 'horizontalAlignment', 'center');
      | 	patch(0,0,[1 1 1]);
      | 	patch(bw,bh,[1 1 1]);
      | else
      | 	tx=bw*0.03;
      | 	ty=bh*0.03;
      | 	patch([0 tx bw bw-tx], [ty 0 bh-ty bh], [1 0 0]);
      | 	patch([0 bw-tx bw tx], [bh-ty 0 ty bh], [1 0 0]);
      | end

== system Model_TranslationEngine64/NEAR/Near1p1/VolumeMute/VolMuteCh4/Ann4NonEntVncApplied/nonentVNCApplied_subsystem ==
  TuneTOP : Subsystem

== system Model_TranslationEngine64/NEAR/Near1p1/VolumeMute/VolMuteCh4/Mute/MuteControl ==
  FeaturePath : FeaturePath/FeaturePath  FeatureName=Ann4Mute  IsGroup=off  GroupNumber=-1  IsModule=off  TriggerInit=[180 39 295 146]
      settings: SourceProductName=Bose Talaria
  TuneVarRampTime : Subsystem  Description=|  mask(Talaria Trivial Tune TOP){TriggerInit=[295 232 465 288], TopName=RampTime, TuneName=RampTime, DataTypeOut=single, MaskValue=Config.DefaultRampTimeMsec, TunabilityNumber=1, MinValue=1, MaxValue=100000, BankNumber=0, PreOverlay=false, PostOverlay=false, UseSameName=on}
      | Specifies the default value of ramp time for the Mute or Unmute operation.
      | Used only when the RTC message does not contain either ramp rate or ramp time.
      mask prompts: TriggerInit "Hidden: MoveFcn redraw"; TopName "Name:"; TuneName "Name of TuneVar:"; DataTypeOut "Data type:"; MaskValue "Default Value:"; TunabilityNumber "Tunability:"; MinValue "Min Value:"; MaxValue "Max Value:"; BankNumber "Target memory bank number:"; PreOverlay "Requires pre-overlay action:"; PostOverlay "Requires post-overlay action:"; UseSameName "Use same name for tune variable and TOP"
      mask help: The TuneTOP block encapsultes a Target Overlay Parameter, a Tune Variable, and a Trivial Translation between them.
      mask init:
      | [ok,activeTopPath,activeTunePath] = TuneTOP_Mask.Init(gcbh);
      settings: MoveFcn=TuneTOP_Mask.CB_TriggerInit(gcbh);
      mask Callback TriggerInit: TuneTOP_Mask.CB_TriggerInit(gcbh);
      mask TypeOptions TopName: TOP/TopName
      mask TypeOptions TuneName: Tune Variable/TuneName
      mask TypeOptions DataTypeOut: TOP/DataTypeOut
      mask TypeOptions MaskValue: Tune Variable/MaskValue
      mask TypeOptions TunabilityNumber: Tune Variable/TunabilityNumber
      mask Callback TunabilityNumber: TuneVarMask.CB_TunabilityNumber(gcbh);
      mask TypeOptions MinValue: Tune Variable/MinValue
      mask TypeOptions MaxValue: Tune Variable/MaxValue
      mask TypeOptions BankNumber: TOP/BankNumber
      mask TypeOptions PreOverlay: TOP/PreOverlay
      mask TypeOptions PostOverlay: TOP/PostOverlay
      mask Callback UseSameName: TuneTOP_Mask.CB_UseSameName(gcbh);
      mask DialogControl toolPanel Prompt: Tuning Tool Hints
      mask DialogControl DescriptionGroup Prompt: Description
      mask DialogControl EditDescription Prompt: Edit Description
      mask DialogControl EditDescription Callback: TuneTOP_Mask.CB_EditDescription(gcbh);
      mask DialogControl TunabilityText Prompt: Easy: Changes nearly every tuning.
      mask DialogControl AdvancedPanel Prompt: Advanced
      mask DialogControl ConvertToFullTranslation Prompt: Irreversible conversion to full translation
      mask DialogControl ConvertToFullTranslation Callback: TuneTOP_Mask.CB_ConvertToFullTranslation(gcbh);
      mask DialogControl ErrorContainer Prompt: Error Messages
      mask Display:
      | % retrieve icon definition
      | [path,w,h] = TuneTOP_Mask.Icon();
      | 
      | % retrieve the block's pixel size
      | pos = get(gcbh,'position');
      | bw = pos(3) - pos(1);
      | bh = pos(4) - pos(2);
      | 
      | % draw centered icon
      | xAdj = bw/2 - w/2 + 5;
      | yAdj = bh/2 - h/2 + 4;
      | for i=1:length(path)
      | 	patch(path(i).x+xAdj, path(i).y+yAdj, path(i).rgb);
      | end
      | 
      | % show the top name or an X
      | if (exist('ok','var') && ok)
      | 	text(bw*0.5, bh*0.2, activeTopPath, 'horizontalAlignment', 'center');
      | 	patch(0,0,[1 1 1]);
      | 	patch(bw,bh,[1 1 1]);
      | else
      | 	tx=bw*0.03;
      | 	ty=bh*0.03;
      | 	patch([0 tx bw bw-tx], [ty 0 bh-ty bh], [1 0 0]);
      | 	patch([0 bw-tx bw tx], [bh-ty 0 ty bh], [1 0 0]);
      | end

== system Model_TranslationEngine64/NEAR/Near1p1/VolumeMute/VolMuteCh4/Volume/TuneVarRampRate ==
  TOP : TOP/TOP  TriggerInit=[440 20 585 80]  TopName=RampRate  DataTypeOut=single  BankNumber=BankNumber  PreOverlay=PreOverlay  PostOverlay=PostOverlay  Role=Automatic
      settings: SourceProductName=Bose Talaria
  TrivialTranslation : TuneVar/TrivialTranslation  TriggerInit=[300 28 350 72]
      settings: SourceProductName=Bose Talaria
  Tune Variable : TuneVar/TuneVar  TuneName=RampRate  SpecifyMaxSize=off  VariableDim=1 (Row)  MaxSize=[1 1]  TunabilityNumber=2  MinValue=MinValue  MaxValue=MaxValue  TriggerInit=[20 25 190 75]  MaskValue=MaskValue
      settings: SourceProductName=Bose Talaria
  wires:
  Tune Variable/1 -> TrivialTranslation/1  "RampRate"
  TrivialTranslation/1 -> TOP/1

== system Model_TranslationEngine64/NEAR/Near1p1/VolumeMute/VolMuteCh4/Volume/TuneVarRampTime ==
  TOP : TOP/TOP  TriggerInit=[440 20 585 80]  TopName=RampTime  DataTypeOut=single  BankNumber=BankNumber  PreOverlay=PreOverlay  PostOverlay=PostOverlay  Role=Automatic
      settings: SourceProductName=Bose Talaria
  TrivialTranslation : TuneVar/TrivialTranslation  TriggerInit=[300 28 350 72]
      settings: SourceProductName=Bose Talaria
  Tune Variable : TuneVar/TuneVar  TuneName=RampTime  SpecifyMaxSize=off  VariableDim=1 (Row)  MaxSize=[1 1]  TunabilityNumber=1  MinValue=MinValue  MaxValue=MaxValue  TriggerInit=[20 25 190 75]  MaskValue=MaskValue
      settings: SourceProductName=Bose Talaria
  wires:
  Tune Variable/1 -> TrivialTranslation/1  "RampTime"
  TrivialTranslation/1 -> TOP/1

== system Model_TranslationEngine64/PostProcess/PostProcess/Mute/Mute/MuteControl/TuneVarRampTime ==
  TOP : TOP/TOP  TriggerInit=[440 20 585 80]  TopName=RampTime  DataTypeOut=single  BankNumber=BankNumber  PreOverlay=PreOverlay  PostOverlay=PostOverlay  Role=Automatic
      settings: SourceProductName=Bose Talaria
  TrivialTranslation : TuneVar/TrivialTranslation  TriggerInit=[300 28 350 72]
      settings: SourceProductName=Bose Talaria
  Tune Variable : TuneVar/TuneVar  TuneName=RampTime  SpecifyMaxSize=off  VariableDim=1 (Row)  MaxSize=[1 1]  TunabilityNumber=1  MinValue=MinValue  MaxValue=MaxValue  TriggerInit=[20 25 190 75]  MaskValue=MaskValue
      settings: SourceProductName=Bose Talaria
  wires:
  Tune Variable/1 -> TrivialTranslation/1  "RampTime"
  TrivialTranslation/1 -> TOP/1

== system Model_TranslationEngine64/ModelPreAmp/DecRate/AudioPilot35/Audiopilot_3_5/ConfigurationRtcInputs/Hvac/table ==
  TOP : TOP/TOP  TriggerInit=[440 20 585 80]  TopName=HvacTable  DataTypeOut=single  BankNumber=0  PreOverlay=false  PostOverlay=false  Role=Automatic
      settings: SourceProductName=Bose Talaria
  TableFormatting : MATLAB Function  TreatAsAtomicUnit=on
  TranslateTrigger : TuneVar/TranslateTrigger  TriggerInit=[306 -100 344 -45]
      settings: SourceProductName=Bose Talaria
  Tune Variable : TuneVar/TuneVar  TuneName=HvacTable  SpecifyMaxSize=on  VariableDim=1 (Row)  MaxSize=[MaskHvacTableSize 2]  TunabilityNumber=1  MinValue=[]  MaxValue=[]  TriggerInit=[20 25 190 75]  MaskValue=Config.HVACTabledBSPL
      settings: SourceProductName=Bose Talaria
  wires:
  TranslateTrigger/1 -> TableFormatting/Trigger
  TableFormatting/1(tableTOP) -> TOP/1
  Tune Variable/1 -> TableFormatting/1(table)  "HvacTable"

== system Model_TranslationEngine64/ModelPreAmp/DecRate/AudioPilot35/Audiopilot_3_5/GainApplication/Compensation/AntizipperRampLpf ==
  Frequency2Coefficients : MATLAB Function  TreatAsAtomicUnit=on
  TOP : TOP/TOP  TriggerInit=[390 20 615 80]  TopName=AntiZipperRampLpfNumerator  DataTypeOut=single  BankNumber=0  PreOverlay=false  PostOverlay=false  Role=Automatic
      settings: SourceProductName=Bose Talaria
  TOP1 : TOP/TOP  TriggerInit=[390 105 615 165]  TopName=AntiZipperRampLpfDenominator  DataTypeOut=Inherit: Same as input  BankNumber=0  PreOverlay=false  PostOverlay=false  Role=Automatic
      settings: SourceProductName=Bose Talaria
  TranslateTrigger : TuneVar/TranslateTrigger  TriggerInit=[256 -100 294 -45]
      settings: SourceProductName=Bose Talaria
  Tune Variable : TuneVar/TuneVar  TuneName=AntiZipperRampFreqHz  SpecifyMaxSize=off  VariableDim=1 (Row)  MaxSize=[1 1]  TunabilityNumber=1  MinValue=[]  MaxValue=[]  TriggerInit=[-85 70 85 120]  MaskValue=Config.AntizipperRampFreqHz
      settings: SourceProductName=Bose Talaria
  wires:
  Tune Variable/1 -> Frequency2Coefficients/1(Freq)  "AntiZipperRampFreqHz"
  Frequency2Coefficients/1(num) -> TOP/1
  TranslateTrigger/1 -> Frequency2Coefficients/Trigger
  Frequency2Coefficients/2(denom) -> TOP1/1

== system Model_TranslationEngine64/ModelPreAmp/DecRate/AudioPilot35/Audiopilot_3_5/GainApplication/Compensation/BassBpf ==
  TOP : TOP/TOP  TriggerInit=[455 -8 670 48]  TopName=BassBpfNumerator  DataTypeOut=single  BankNumber=0  PreOverlay=false  PostOverlay=false  Role=Automatic
      settings: SourceProductName=Bose Talaria
  TOP1 : TOP/TOP  TriggerInit=[455 60 670 120]  TopName=BassBpfDenominator  DataTypeOut=single  BankNumber=0  PreOverlay=false  PostOverlay=false  Role=Automatic
      settings: SourceProductName=Bose Talaria
  TranslateTrigger : TuneVar/TranslateTrigger  TriggerInit=[306 -100 344 -45]
      settings: SourceProductName=Bose Talaria
  Tune Variable : TuneVar/TuneVar  TuneName=BassBpfCenterFreqHz  SpecifyMaxSize=off  VariableDim=1 (Row)  MaxSize=[1 1]  TunabilityNumber=1  MinValue=[]  MaxValue=[]  TriggerInit=[-55 -5 115 45]  MaskValue=Config.BassBpfCenterFreqHz
      settings: SourceProductName=Bose Talaria
  Tune Variable1 : TuneVar/TuneVar  TuneName=BassBpfQ  SpecifyMaxSize=off  VariableDim=1 (Row)  MaxSize=[1 1]  TunabilityNumber=1  MinValue=[]  MaxValue=[]  TriggerInit=[-55 65 115 115]  MaskValue=Config.BassBpfQ
      settings: SourceProductName=Bose Talaria
  wcQ2coefs : MATLAB Function  TreatAsAtomicUnit=on
  wires:
  Tune Variable/1 -> wcQ2coefs/1(freq)  "BassBpfCenterFreqHz"
  wcQ2coefs/1(num) -> TOP/1
  TranslateTrigger/1 -> wcQ2coefs/Trigger
  wcQ2coefs/2(denom) -> TOP1/1
  Tune Variable1/1 -> wcQ2coefs/2(Qin)  "BassBpfQ"
